simulink model "psbdcmotor"  (Simulink 6.0)
settings: Solver=ode23s  SolverMode=SingleTasking  StartTime=0.0  StopTime=10  RelTol=1e-3  AbsTol=1e-2
libraries: powerlib2 x20, powerlib_extras x1, simulink x1
settings Model: Creator=patrice  LastModifiedBy=batserve  ExtModeTrigMode=oneshot  ExtModeArmWhenConnect=off  ExtModeAutoUpdateStatusClock=off
settings DataIOCC: Decimation=5  FinalStateName=x50  InitialState=x50  LimitDataPoints=off  MaxDataPoints=500000  SaveOutput=off  TimeSaveName=t  SignalLoggingName=sigsOut
settings OptimizationCC: BlockReduction=off  BooleanDataType=off
settings DebuggingCC: CheckExecutionContextPreStartOutputMsg=on  CheckExecutionContextRuntimeOutputMsg=on  SolverPrmCheckMsg=none  IntegerOverflowMsg=none
settings HardwareCC: TargetUnknown=on
settings RTWCC: TemplateMakefile=grt_vc.tmf

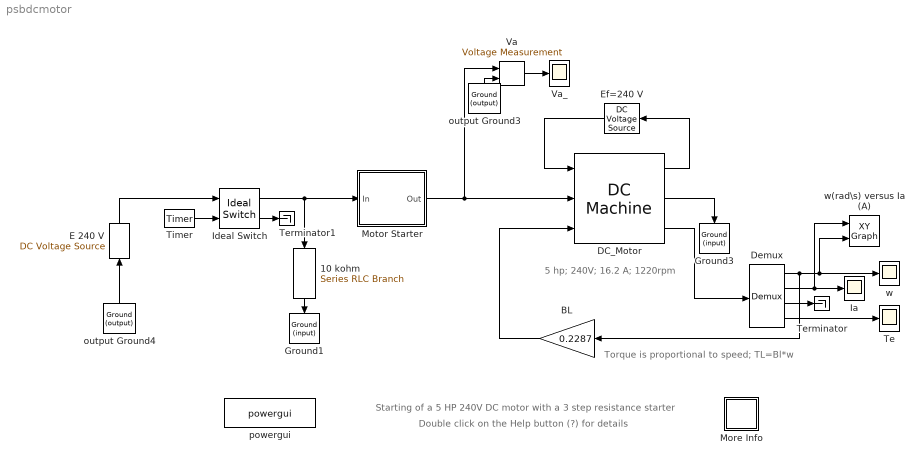
== system psbdcmotor ==
  note: Starting of a 5 HP 240V DC motor with a 3 step resistance starter
  note: 5 hp; 240V; 16.2 A; 1220rpm
  note: Torque is proportional to speed; TL=Bl*w
  note: Double click on the Help button (?) for details
  10 kohm : powerlib2/Elements/Series RLC Branch  Tag=PoWeRsYsTeMbLoCk  Orientation=down  a=1e4  b=0  c=inf  mesure=None  PSBOutputType=1
  BL : Gain  Orientation=left  Gain=0.2287  SaturateOnIntegerOverflow=on
  DC_Motor : powerlib2/Machines/DC Machine  RLa="[ 0.6  0.012]"  RLf="[ 240  120]"  Laf=1.8  J=1  Bm=0  Tf=0  w0=1  PSBOutputType=110
  Demux : Demux
  E 240 V : powerlib2/Electrical Sources/DC Voltage Source  Tag=PoWeRsYsTeMbLoCk  Orientation=up  V=240  mesure=None  PSBOutputType=1
  Ef=240 V : powerlib2/Electrical Sources/DC Voltage Source  Tag=PoWeRsYsTeMbLoCk  Orientation=left  V=240  mesure=None  PSBOutputType=1
  Ground1 : powerlib2/Connectors/Ground (input)  Tag=PoWeRsYsTeMbLoCk  Orientation=down
  Ground3 : powerlib2/Connectors/Ground (input)  Tag=PoWeRsYsTeMbLoCk  Orientation=down
  Ia : Scope
      settings: TickLabels=on  TimeRange=10  YMin=0  YMax=40  SaveName=Ia  DataFormat=Array  MaxDataPoints=500000
  Ideal Switch : powerlib2/Power Electronics/Ideal Switch  Tag=PoWeRsYsTeMbLoCk  Ron=1e-4  Lon=10e-6  IC=0  Rs=inf  Cs=0  PSBOutputType=10
  More Info : Subsystem
      mask Display: disp('?')
  Motor Starter : Subsystem
      mask Display: disp('3 step\n\nstarter')
  Te : Scope
      settings: TickLabels=on  TimeRange=10  YMin=0  YMax=100  SaveName=Tm  DataFormat=Array  MaxDataPoints=500000
  Terminator : Terminator
  Terminator1 : Terminator
  Timer : powerlib_extras/Control  Blocks/Timer  t=[0 0.5 ]  e=[0 1 ]
  Va : powerlib2/Measurements/Voltage Measurement  Tag=PoWeRsYsTeMmEaSuReMeNt  PhasorSimulation=off  OutputType=Magnitude  PSBOutputType=0  PSBequivalent=0
  Va_ : Scope
      settings: TickLabels=on  TimeRange=10  YMin=0  YMax=300  SaveName=U_DC_mot  DataFormat=Array  MaxDataPoints=500000
  output Ground3 : powerlib2/Connectors/Ground (output)  Tag=PoWeRsYsTeMbLoCk  Orientation=up  PSBOutputType=1
  output Ground4 : powerlib2/Connectors/Ground (output)  Tag=PoWeRsYsTeMbLoCk  Orientation=up  PSBOutputType=1
  powergui : powerlib2/powergui  Frange=logspace(0,3,50)  Ylog=off  Xlog=off  save=off  variable=ZData  ZoomFFT=on  StartTime=0.0  cycles=1  DisplayStyle=off  fundamental=60  FreqAxis=off  MaxFrequency=1000  frequencyindice=1  frequencyindicesteady=1  RmsSteady=1  display=off  Ts=0  methode=off  frequency=60  echomessages=off
  w : Scope
      settings: TickLabels=on  TimeRange=10  YMin=0  YMax=150  SaveName=w  DataFormat=Array  MaxDataPoints=500000
  w(rad\s) versus Ia (A) : simulink/Sinks/XY Graph  xmin=0  xmax=40  ymin=0  ymax=140  st=-1
  wires:
  Timer/1 -> Ideal Switch/2
  output Ground4/1 -> E 240 V/1
  10 kohm/1 -> Ground1/1
  DC_Motor/3 -> Demux/1
  Demux/4 -> Te/1
  Ideal Switch/1 -> 10 kohm/1, Motor Starter/1(In)
  E 240 V/1 -> Ideal Switch/1
  Demux/1 -> BL/1, w/1, w(rad\s) versus Ia (A)/2
  BL/1 -> DC_Motor/3
  Demux/2 -> Ia/1, w(rad\s) versus Ia (A)/1
  Motor Starter/1(Out) -> Va/1, DC_Motor/2
  DC_Motor/2 -> Ground3/1
  output Ground3/1 -> Va/2
  Va/1 -> Va_/1
  Ef=240 V/1 -> DC_Motor/1
  DC_Motor/1 -> Ef=240 V/1
  Demux/3 -> Terminator/1
  Ideal Switch/2 -> Terminator1/1

== system psbdcmotor/More Info ==
  note: Induced EMF:  Eo-=240-16.2*0.6=230.3 V
      |
      | Pe = 230.3*16.2=3731 W = 5.0 HP
      |
      | Field current: If = 240/240 =1 A
      |
      | Eo = w*Laf*If  --->  w = (Eo/La*If)
      | speed w = 230.3/1.8 = 127.7 rad/s = 1220 r/min
      |
      | Nominal  torque: Te = Pe/w = 3731/127.7 = 29.2 N.m
  note: DC Motor Rated Values:
  note: (Krause et al., Reference Analysis of Electric Machinery, pp 89-92)
  note: Starting a 5 HP, 240V DC motor with a 3-step resistance starter
  note: G. Sybille (Hydro-Quebec)

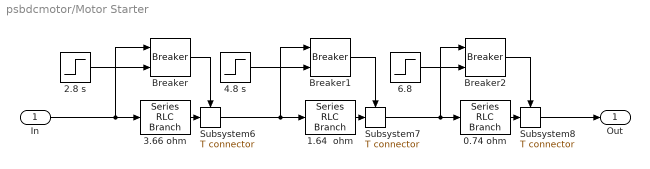
== system psbdcmotor/Motor Starter ==
  In : Inport  Port=1  LatchInput=off
  0.74 ohm : powerlib2/Elements/Series RLC Branch  Tag=PoWeRsYsTeMbLoCk  a=0.74  b=0  c=inf  mesure=None  PSBOutputType=1
  1.64  ohm : powerlib2/Elements/Series RLC Branch  Tag=PoWeRsYsTeMbLoCk  a=1.64  b=0  c=inf  mesure=None  PSBOutputType=1
  2.8 s : Step  Time=2.8  SampleTime=0  ZeroCross=off
  3.66 ohm : powerlib2/Elements/Series RLC Branch  Tag=PoWeRsYsTeMbLoCk  a=3.66  b=0  c=inf  mesure=None  PSBOutputType=1
  4.8 s : Step  Time=4.8  SampleTime=0  ZeroCross=off
  6.8 : Step  Time=6.8  SampleTime=0  ZeroCross=off
  Breaker : powerlib2/Elements/Breaker  Tag=PoWeRsYsTeMbLoCk  a=0.01  c=0  rs=inf  cs=0  times="[ 4/60  5/60 ]"  Ts=0  comext=on  mesure=None  PSBOutputType=1
  Breaker1 : powerlib2/Elements/Breaker  Tag=PoWeRsYsTeMbLoCk  a=0.01  c=0  rs=inf  cs=0  times="[ 4/60  5/60 ]"  Ts=0  comext=on  mesure=None  PSBOutputType=1
  Breaker2 : powerlib2/Elements/Breaker  Tag=PoWeRsYsTeMbLoCk  a=0.01  c=0  rs=inf  cs=0  times="[ 4/60  5/60 ]"  Ts=0  comext=on  mesure=None  PSBOutputType=1
  Subsystem6 : powerlib2/Connectors/T connector  Tag=PoWeRsYsTeMbLoCk  PSBOutputType=1
  Subsystem7 : powerlib2/Connectors/T connector  Tag=PoWeRsYsTeMbLoCk  PSBOutputType=1
  Subsystem8 : powerlib2/Connectors/T connector  Tag=PoWeRsYsTeMbLoCk  PSBOutputType=1
  Out : Outport  InitialOutput=0
  wires:
  In/1 -> 3.66 ohm/1, Breaker/1
  3.66 ohm/1 -> Subsystem6/1
  Breaker/1 -> Subsystem6/Enable
  1.64  ohm/1 -> Subsystem7/1
  Breaker1/1 -> Subsystem7/Enable
  Subsystem6/1 -> 1.64  ohm/1, Breaker1/1
  0.74 ohm/1 -> Subsystem8/1
  Breaker2/1 -> Subsystem8/Enable
  Subsystem7/1 -> 0.74 ohm/1, Breaker2/1
  Subsystem8/1 -> Out/1
  4.8 s/1 -> Breaker1/2
  6.8/1 -> Breaker2/2
  2.8 s/1 -> Breaker/2
